simulink model "model"  (R2020b)
settings: Solver=VariableStepAuto  StartTime=0.0  StopTime=10.0  RelTol=1e-3
settings Model: Creator=Vrunda M Balgi  LastModifiedBy=Vrunda M Balgi

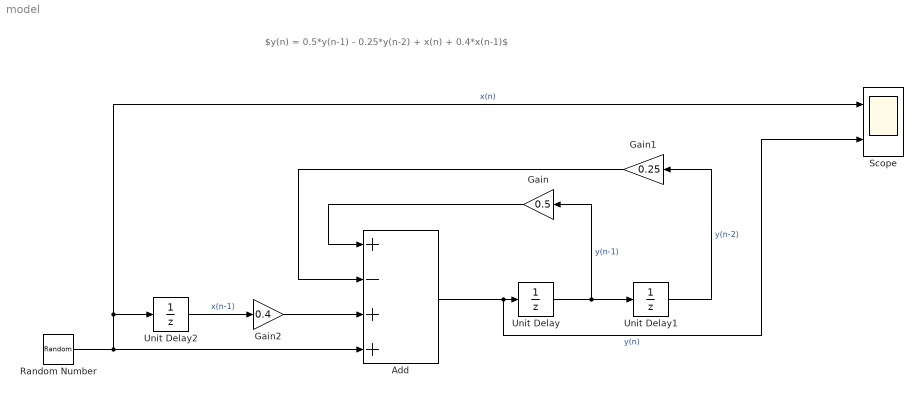
== system model ==
  note: $y(n) = 0.5*y(n-1) - 0.25*y(n-2) + x(n) + 0.4*x(n-1)$
  Add : Sum  Inputs=+-++
  Gain : Gain  Gain=0.5
  Gain1 : Gain  Gain=0.25
  Gain2 : Gain  Gain=0.4
  Random Number : RandomNumber  SampleTime=0.1
  Scope : Scope  NumInputPorts=2
  Unit Delay : UnitDelay  SampleTime=-1  HasFrameUpgradeWarning=on
  Unit Delay1 : UnitDelay  SampleTime=-1  HasFrameUpgradeWarning=on
  Unit Delay2 : UnitDelay  SampleTime=-1  HasFrameUpgradeWarning=on
  wires:
  Add/1 -> Scope/2, Unit Delay/1  "y(n)"
  Unit Delay/1 -> Gain/1, Unit Delay1/1  "y(n-1)"
  Unit Delay1/1 -> Gain1/1  "y(n-2)"
  Gain/1 -> Add/1
  Gain1/1 -> Add/2
  Random Number/1 -> Unit Delay2/1, Scope/1, Add/4  "x(n)"
  Unit Delay2/1 -> Gain2/1  "x(n-1)"
  Gain2/1 -> Add/3
